simulink model "linear_sys"  (R2017a)
settings: Solver=VariableStepAuto  StartTime=0.0  StopTime=10.0  RelTol=1e-3
undefined symbols (not defined in the file or in its folder): DC, NC
settings Model: Creator=julio  LastModifiedBy=julio

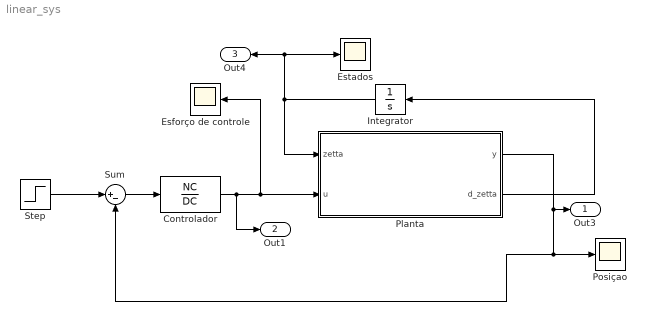
== system linear_sys ==
  Controlador : TransferFcn  Numerator=NC  Denominator=DC  ContinuousStateAttributes='Controler'
  Esforço de controle : Scope
  Estados : Scope
  Integrator : Integrator  InitialCondition=[0 0 0 0]
  Planta : MATLAB Function  TreatAsAtomicUnit=on  RTWFcnName=linear_func  RTWFileName=linear_func
      settings: MinAlgLoopOccurrences=on  RTWFileNameOpts=User specified
  Posiçao : Scope
  Step : Step  Time=0  After=10  SampleTime=0
  Sum : Sum  Inputs=|+-
  Out3 : Outport  SignalName=y
  Out1 : Outport  Port=2  SignalName=esf
  Out4 : Outport  Port=3  SignalName=state
  wires:
  Planta/1(y) -> Out3/1, Sum/2, Posiçao/1
  Sum/1 -> Controlador/1
  Controlador/1 -> Out1/1, Planta/2(u), Esforço de controle/1
  Step/1 -> Sum/1
  Integrator/1 -> Planta/1(zetta), Estados/1, Out4/1
  Planta/2(d_zetta) -> Integrator/1

== matlab function linear_sys/Planta ==
  data: zetta input size=4; u input size=1; y output size=1; d_zetta output size=4
function [ y, d_zetta] = linear_func( zetta, u )
%LINEAR_FUNC Summary of this function goes here
%   Detailed explanation goes here
    MJ = 1.0731; % [kg]
    m  = 0.209;  % [kg]
    l  = 0.3302; % [m]
    bK = 5.4;    % [N.s/(m²)]
    Kr = 1.0717; % [N/V]
    g  = 9.81;   % [m/s²]
    
    A = [0 1 0 0
        0 -bK/MJ m*g/MJ 0
        0 0 0 1
        0 bK/(MJ*l) -((g/l)+(m*g/(MJ*l))) 0];
    
    B = [0 
        Kr/MJ
        0
        -Kr/(MJ*l)];
    
    C = [1 0 0 0];
    
    D = [0];
    
    d_zetta = A*zetta + B*u;
    
    y = C*zetta + D*u;
end
